simulink library "Body_CAD"  (R2026a)
settings: Solver=VariableStepAuto
undefined symbols (not defined in the file): BodyGeometry, X, Y, Z
libraries: sm_lib x2
Description:
  | Component of Simscape Vehicle Templates Library
  | 
  | Copyright 2018-2026 The MathWorks, Inc.
settings Model: Creator=smiller  LastModifiedBy=smiller

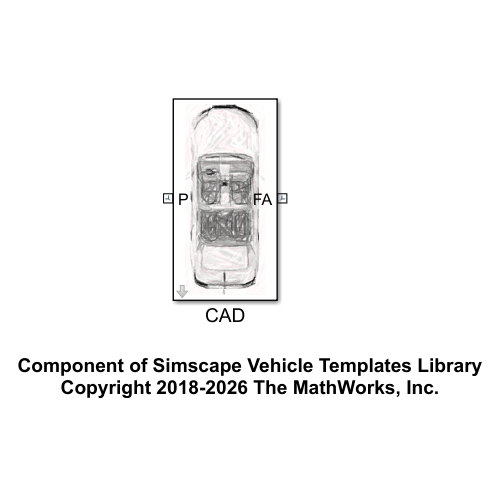
[thumbnail: Simulink's stored preview of the top-level diagram]
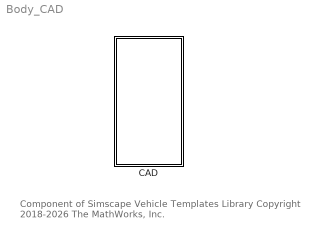
== system Body_CAD ==
  note: Component of Simscape Vehicle Templates Library
      | Copyright 2018-2026 The MathWorks, Inc.
  CAD : Subsystem  mask(Body Geometry from CAD){cad_file=BodyGeometry.filename.Value, cad_units=BodyGeometry.fileunits.Value, cad_xyz=BodyGeometry.sOffset.Value, cad_ypr=BodyGeometry.aOffset.Value, cad_clr=BodyGeometry.Color.Value, cad_opc=BodyGeometry.Opacity.Value}
      mask prompts: cad_file "CAD File"; cad_units "Units"; cad_xyz "Offset to reference [xyz] (m)"; cad_ypr "Offset yaw-pitch-roll  (rad)"; cad_clr "Color [RGB]"; cad_opc "Opacity (0-1)"
      mask help: Specify vehicle body geometry from a single CAD file.
      mask init:
      | set_param([gcb '/Geometry'],'ExtGeomFileName',cad_file);
      | set_param([gcb '/Geometry'],'ExtGeomFileUnits',cad_units);
      mask Display: image('sm_car_bodygeometry_cad.png');

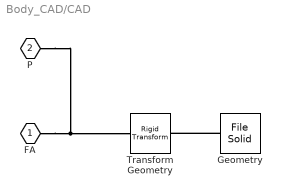
== system Body_CAD/CAD ==
  Geometry : sm_lib/Body Elements/File Solid  ExtGeomFileName=Sedan_CAD.stl  UnitType=Custom  ExtGeomFileUnits=m  StepReaderType=HEX  ExportConvexHullGeometry=off  InertiaType=Custom  BasedOnType=DensityFromFile  Density=1000  DensityUnits=kg/m^3  Mass=1  MassUnits=kg  CenterOfMass=[0 0 0]  CenterOfMassUnits=m  MomentsOfInertia=[1 1 1]  MomentsOfInertiaUnits=kg*m^2  ProductsOfInertia=[0 0 0]  ProductsOfInertiaUnits=kg*m^2  GraphicType=FromGeometry  MarkerShape=Sphere  MarkerSize=10  GraphicVisPropType=SimpleVisualProperties  GraphicDiffuseColor=cad_clr  GraphicOpacity=cad_opc  GraphicSpecularColor=[0.5 0.5 0.5 1.0]  GraphicAmbientColor=[0.15 0.15 0.15 1.0]  GraphicEmissiveColor=[0.0 0.0 0.0 1.0]  GraphicShininess=75  DoExposeReferenceFrame=on  SerializedFrames=<Frames/>
  Transform Geometry : sm_lib/Frames and Transforms/Rigid Transform  RotationMethod=RotationSequence  FollAlignAxisA=+X  BaseAlignAxisA=+Y  FollAlignAxisB=+Y  BaseAlignAxisB=+Z  RotationStandardAxis=+Z  RotationAngle=0  RotationAngleUnits=rad  RotationArbitraryAxis=[0 0 1]  RotationSequenceAxes=FollowerAxes  RotationSequence=ZYX  RotationSequenceAngles=cad_ypr  RotationSequenceAnglesUnits=rad  RotationMatrix=[1 0 0; 0 1 0; 0 0 1]  Quaternion=[1 0 0 0]  TranslationMethod=Cartesian  TranslationCartesianOffset=cad_xyz  TranslationCartesianOffsetUnits=m  TranslationStandardAxis=+Z  TranslationStandardOffset=0  TranslationStandardOffsetUnits=m  TranslationROffset=0  TranslationROffsetUnits=m  TranslationThetaOffset=0  TranslationThetaOffsetUnits=deg  TranslationZOffset=0  TranslationZOffsetUnits=m
  FA : PMIOPort  Side=Right
  P : PMIOPort  Port=2  Side=Left
  connections:
  Geometry/RConn1 -- Transform Geometry/RConn1
  FA/RConn1 -- P/RConn1 -- Transform Geometry/LConn1
